simulink model "pro1_21011324"  (R2024b)
settings: Solver=VariableStepAuto  StartTime=0.0  StopTime=500  RelTol=1e-3
InitFcn:
  | %% environment Parameter
  | 
  | g = 9.8066;                      %[m s^2]
  | 
  | %% vehicle Parameter
  | 
  | mass = 1.5;                     %[N]
  | Arm_Length = 0.225;              %[m]
  | %% Motor Parameter
  | 
  | rpm2rad = 2 * pi/60 ;
  | rad2rpm = 1 / rpm2rad;
  | 
  | Friction_Coef = 0.0001;         %[N m/s]
  | Inertia = 2.8e-05;              %[kg m^2]
  | Resistance = 0.1170;            %[ohm]
  | K_Torque = 1 / (rpm2rad * 960); %[N m/A]
  | K_Emf = K_Torque;               %[V s/rad]
  | 
  | Tau = (Inertia * Resistance) / (Resistance * Friction_Coef + K_Torque * K_Emf);
  | 
  | ks = K_Torque / (Resistance * Friction_Coef + K_Torque * K_Emf);
  | 
  | Trust_Coef = 1.1768e-05;        %[N s^2]
  | Drag_Coef = 1.8542e-07;         %[N  m s^2]
  | Hovering_Speed = sqrt((mass * g)/(4 * Trust_Coef));
  | 
  | kp = 0.011;
  | 
  | K1_ALT = 2.1;
  | K2_ALT = 0.7142;
  | 
  | K1_POS = 1.26;
  | K2_POS = 0.4286;
  | 
  | 
  | %waypoint flight
  | wp_1=[0; 0; 80];     %충무관 [m]
  | wp_2=[-564.04; -102.42; 80 ]; % 순리[m]
  | wp_3=[-3714.7; 689.55; 80]; %잠실유람선터미널 [m]
  | wp_home=[0; 0; 50];
libraries: simulink_extras x2, simulink x1, hdlsllib x1
settings Model: Creator=정욱  LastModifiedBy=HOME
settings ConfigComp: CovBoundaryAbsTol=1.0e-5

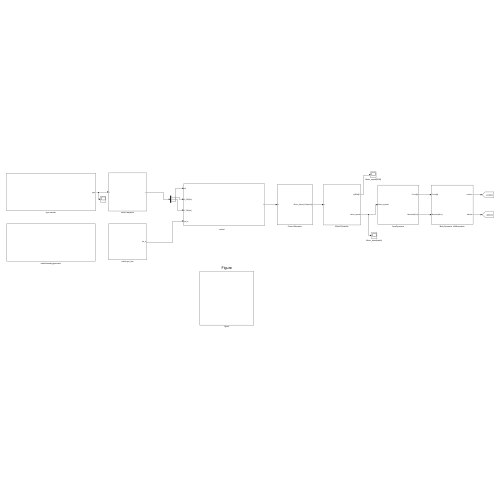
[thumbnail: Simulink's stored preview of the top-level diagram]
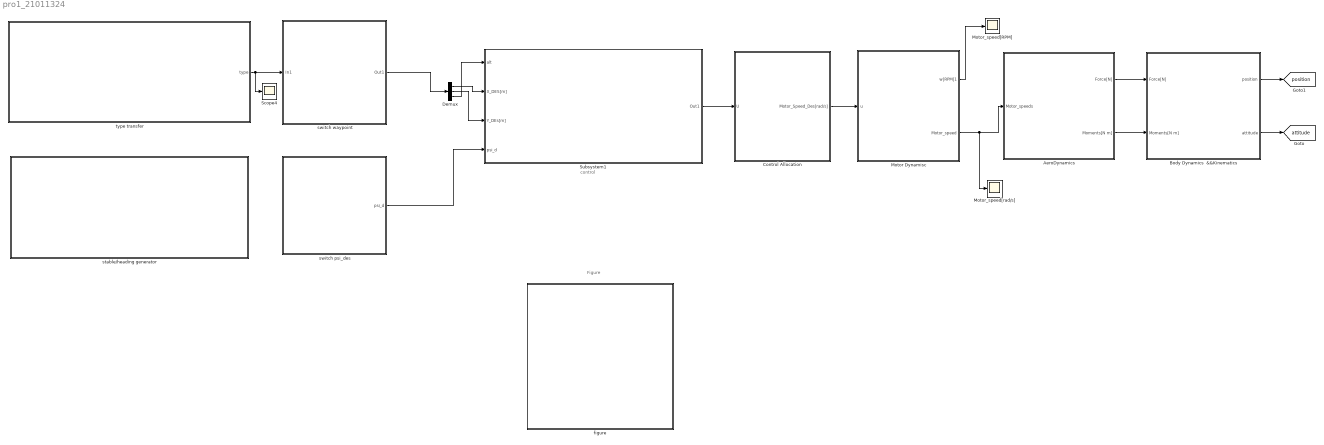
== system pro1_21011324 ==
  note: Figure
  note: control
  AeroDynamics : Subsystem
  Body Dynamics  &&Kinematics : Subsystem
  Control Allocation : Subsystem
  Demux : Demux  Outputs=3
  Motor Dynamisc : Subsystem
  Motor_speed[RPM] : Scope
  Motor_speed[rad/s] : Scope
  Scope4 : Scope
  Subsystem1 : Subsystem
  figure : Subsystem
  stable/heading generator : Subsystem
  switch psi_des : Subsystem
  switch waypoint : Subsystem
  type transfer : Subsystem
  tag scope: attitude=global, position=global
  wires:
  Motor Dynamisc/1(w[RPM]1) -> Motor_speed[RPM]/1
  Motor Dynamisc/2(Motor_speed) -> AeroDynamics/1(Motor_speeds), Motor_speed[rad/s]/1
  Body Dynamics  &&Kinematics/2(attitude) -> [attitude]
  Body Dynamics  &&Kinematics/1(position) -> [position]
  AeroDynamics/1(Force[N]) -> Body Dynamics  &&Kinematics/1(Force[N])
  AeroDynamics/2(Moments[N m]) -> Body Dynamics  &&Kinematics/2(Moments[N m])
  Control Allocation/1(Motor_Speed_Des[rad/s]) -> Motor Dynamisc/1(u)
  Subsystem1/1(Out1) -> Control Allocation/1(U)
  Demux/1 -> Subsystem1/2(X_DES[m])
  Demux/2 -> Subsystem1/3(Y_DEs[m])
  Demux/3 -> Subsystem1/1(alt)
  type transfer/1(type) -> Scope4/1, switch waypoint/1(In1)
  switch waypoint/1(Out1) -> Demux/1
  switch psi_des/1(psi_d) -> Subsystem1/4(psi_d)

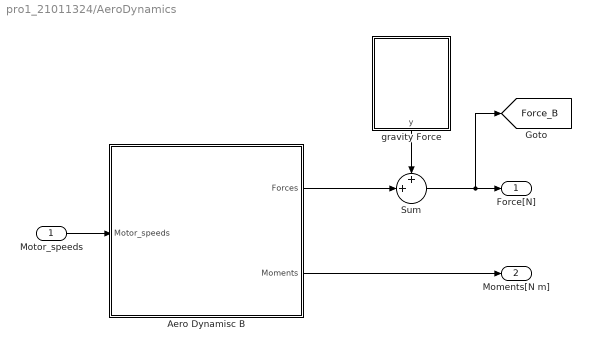
== system pro1_21011324/AeroDynamics ==
  Motor_speeds : Inport
  Aero Dynamisc B : MATLAB Function  TreatAsAtomicUnit=on
  Sum : Sum  Inputs=++|
  "gravity Force " : Subsystem
  Force[N] : Outport
  Moments[N m] : Outport  Port=2
  tag scope: Force_B=global
  wires:
  Aero Dynamisc B/1(Forces) -> Sum/2
  "gravity Force "/1(y) -> Sum/1
  Aero Dynamisc B/2(Moments) -> Moments[N m]/1
  Motor_speeds/1 -> Aero Dynamisc B/1(Motor_speeds)
  Sum/1 -> Force[N]/1, [Force_B]

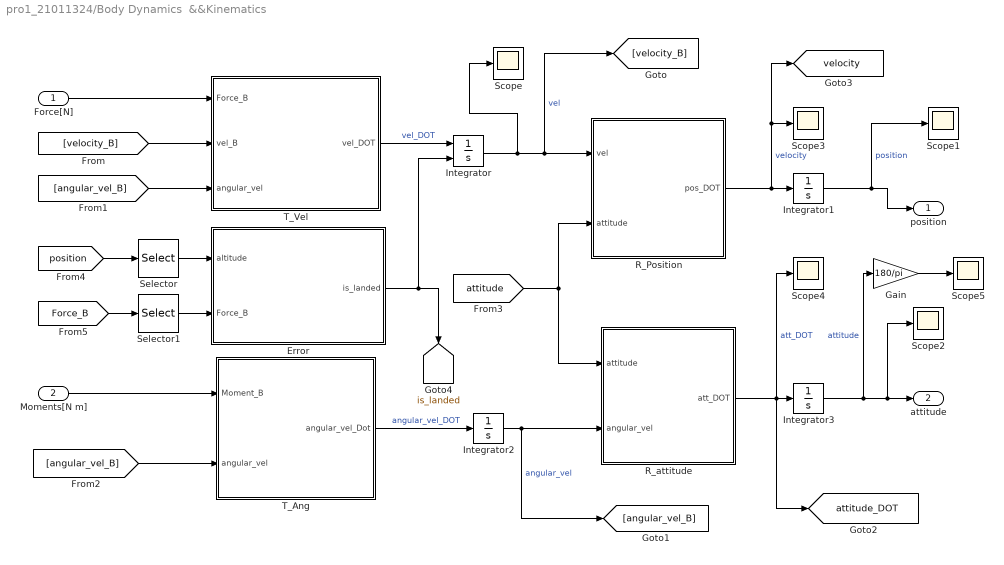
== system pro1_21011324/Body Dynamics  &&Kinematics ==
  Force[N] : Inport
  Moments[N m] : Inport  Port=2
  Error : MATLAB Function  TreatAsAtomicUnit=on
  Gain : Gain  Gain=180/pi
  Integrator : Integrator  ExternalReset=level hold  InitialCondition=[0;0;0]
  Integrator1 : Integrator  InitialCondition=[0;0;0]  LimitOutput=on  UpperSaturationLimit=[inf;inf;0]  LowerSaturationLimit=[-inf;-inf;-inf]  ZeroCross=off
  Integrator2 : Integrator  InitialCondition=[0;0;0]
  Integrator3 : Integrator  InitialCondition=[0;0;0]  WrapState=on
  R_Position : MATLAB Function  TreatAsAtomicUnit=on
  R_attitude : MATLAB Function  TreatAsAtomicUnit=on
  Scope{,1..5} (6 alike) : Scope
  Selector : Selector  InputPortWidth=3  IndexOptions=Index vector (dialog)  Indices=[3]  OutputSizes=1
  Selector1 : Selector  InputPortWidth=3  IndexOptions=Index vector (dialog)  Indices=[3]  OutputSizes=1
  T_Ang : MATLAB Function  TreatAsAtomicUnit=on
  T_Vel : MATLAB Function  TreatAsAtomicUnit=on
  position : Outport
  attitude : Outport  Port=2
  tag scope: attitude_DOT=global, is_landed=global, velocity=global
  wires:
  Force[N]/1 -> T_Vel/1(Force_B)
  Moments[N m]/1 -> T_Ang/1(Moment_B)
  T_Vel/1(vel_DOT) -> Integrator/1  "vel_DOT"
  Integrator/1 -> [velocity_B], R_Position/1(vel), Scope/1  "vel"
  R_Position/1(pos_DOT) -> [velocity], Scope3/1, Integrator1/1  "velocity"
  Integrator1/1 -> Scope1/1, position/1  "position"
  T_Ang/1(angular_vel_Dot) -> Integrator2/1  "angular_vel_DOT"
  Integrator2/1 -> R_attitude/2(angular_vel), [angular_vel_B]  "angular_vel"
  R_attitude/1(att_DOT) -> Scope4/1, [attitude_DOT], Integrator3/1  "att_DOT"
  Integrator3/1 -> Gain/1, Scope2/1, attitude/1  "attitude"
  [velocity_B] -> T_Vel/2(vel_B)
  [angular_vel_B] -> T_Vel/3(angular_vel)
  [angular_vel_B] -> T_Ang/2(angular_vel)
  [attitude] -> R_Position/2(attitude), R_attitude/1(attitude)
  [position] -> Selector/1
  [Force_B] -> Selector1/1
  Selector1/1 -> Error/2(Force_B)
  Selector/1 -> Error/1(altitude)
  Error/1(is_landed) -> [is_landed], Integrator/2
  Gain/1 -> Scope5/1

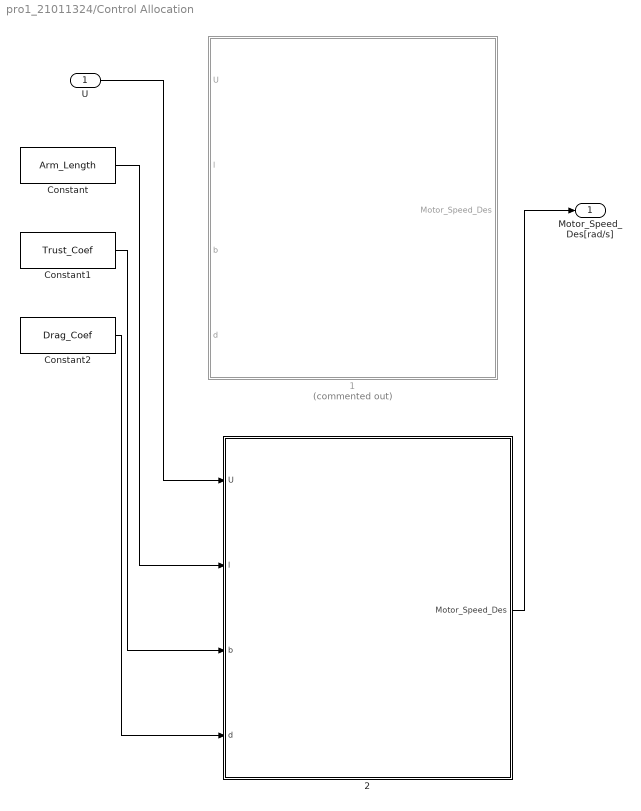
== system pro1_21011324/Control Allocation ==
  U : Inport
  1 : MATLAB Function  Commented=on  TreatAsAtomicUnit=on
  2 : MATLAB Function  TreatAsAtomicUnit=on
  Constant : Constant  Value=Arm_Length
  Constant1 : Constant  Value=Trust_Coef
  Constant2 : Constant  Value=Drag_Coef
  Motor_Speed_Des[rad/s] : Outport
  wires:
  U/1 -> 2/1(U)
  Constant/1 -> 2/2(l)
  Constant1/1 -> 2/3(b)
  Constant2/1 -> 2/4(d)
  2/1(Motor_Speed_Des) -> Motor_Speed_Des[rad/s]/1

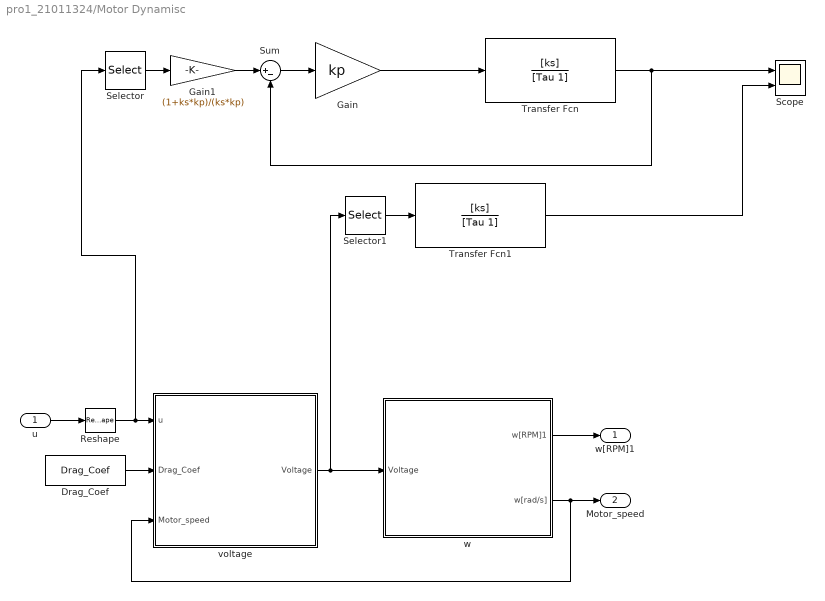
== system pro1_21011324/Motor Dynamisc ==
  u : Inport
  Drag_Coef : Constant  Value=Drag_Coef
  Gain : Gain  Gain=kp
  Gain1 : Gain  Gain=(1+ks*kp)/(ks*kp)
  Reshape : Reshape  OutputDimensionality=Column vector (2-D)
  Scope : Scope  NumInputPorts=2
  Selector : Selector  InputPortWidth=4  IndexOptions=Index vector (dialog)  Indices=1  OutputSizes=1
  Selector1 : Selector  InputPortWidth=4  IndexOptions=Index vector (dialog)  Indices=1  OutputSizes=1
  Sum : Sum  Inputs=|+-
  Transfer Fcn : TransferFcn  Numerator=[ks]  Denominator=[Tau 1]
  Transfer Fcn1 : TransferFcn  Numerator=[ks]  Denominator=[Tau 1]
  voltage : MATLAB Function  TreatAsAtomicUnit=on
  w : Subsystem
  w[RPM]1 : Outport
  Motor_speed : Outport  Port=2
  wires:
  voltage/1(Voltage) -> Selector1/1, w/1(Voltage)
  w/2(w[rad/s]) -> voltage/3(Motor_speed), Motor_speed/1
  u/1 -> Reshape/1
  Drag_Coef/1 -> voltage/2(Drag_Coef)
  w/1(w[RPM]1) -> w[RPM]1/1
  Reshape/1 -> Selector/1, voltage/1(u)
  Selector1/1 -> Transfer Fcn1/1
  Sum/1 -> Gain/1
  Gain/1 -> Transfer Fcn/1
  Transfer Fcn/1 -> Scope/1, Sum/2
  Transfer Fcn1/1 -> Scope/2
  Gain1/1 -> Sum/1
  Selector/1 -> Gain1/1

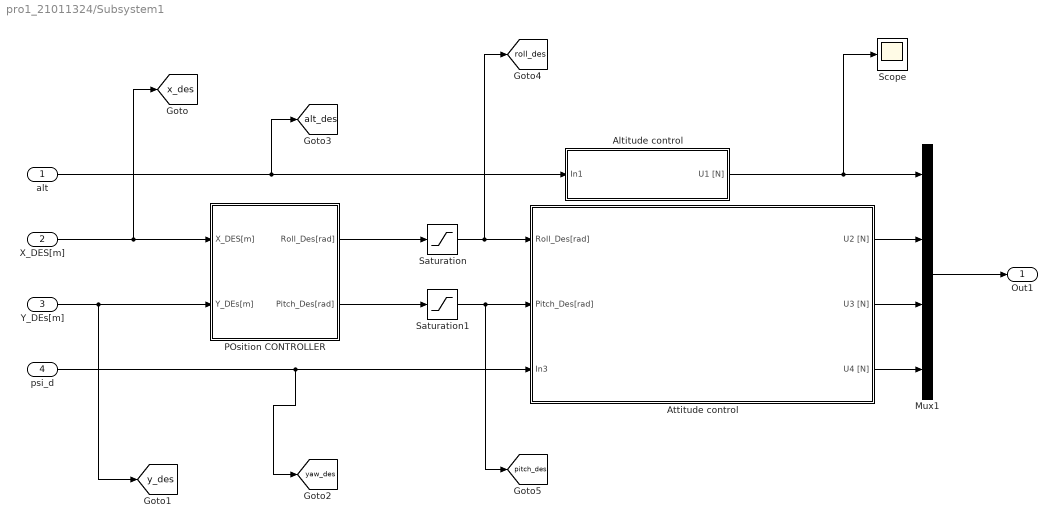
== system pro1_21011324/Subsystem1 ==
  alt : Inport
  X_DES[m] : Inport  Port=2
  Y_DEs[m] : Inport  Port=3
  psi_d : Inport  Port=4
  Altitude control : Subsystem
  Attitude control : Subsystem
  Mux1 : Mux
  POsition CONTROLLER : Subsystem
  Saturation : Saturate  UpperLimit=deg2rad(30)  LowerLimit=-deg2rad(30)
  Saturation1 : Saturate  UpperLimit=deg2rad(30)  LowerLimit=-deg2rad(30)
  Scope : Scope
  Out1 : Outport
  tag scope: alt_des=global, pitch_des=global, roll_des=global, x_des=global, y_des=global, yaw_des=global
  wires:
  Attitude control/3(U4 [N]) -> Mux1/4
  Attitude control/1(U2 [N]) -> Mux1/2
  Saturation/1 -> [roll_des], Attitude control/1(Roll_Des[rad])
  Altitude control/1(U1 [N]) -> Scope/1, Mux1/1
  POsition CONTROLLER/1(Roll_Des[rad]) -> Saturation/1
  Saturation1/1 -> [pitch_des], Attitude control/2(Pitch_Des[rad])
  POsition CONTROLLER/2(Pitch_Des[rad]) -> Saturation1/1
  Attitude control/2(U3 [N]) -> Mux1/3
  Y_DEs[m]/1 -> POsition CONTROLLER/2(Y_DEs[m]), [y_des]
  psi_d/1 -> [yaw_des], Attitude control/3(In3)
  X_DES[m]/1 -> POsition CONTROLLER/1(X_DES[m]), [x_des]
  alt/1 -> [alt_des], Altitude control/1(In1)
  Mux1/1 -> Out1/1

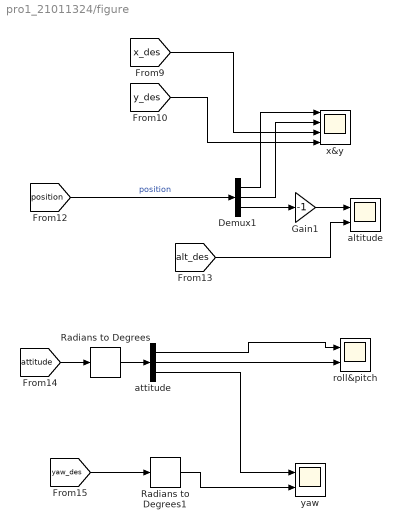
== system pro1_21011324/figure ==
  Demux1 : Demux  Outputs=3
  Gain1 : Gain  Gain=-1
  Radians to Degrees : simulink_extras/Transformations/Radians to Degrees
  Radians to Degrees1 : simulink_extras/Transformations/Radians to Degrees
  altitude : Scope  NumInputPorts=2
  attitude : Demux  Outputs=3
  roll&pitch : Scope  NumInputPorts=2
  x&y : Scope  NumInputPorts=4
  yaw : Scope  NumInputPorts=2
  wires:
  [position] -> Demux1/1  "position"
  Gain1/1 -> altitude/1
  [attitude] -> Radians to Degrees/1
  Demux1/2 -> x&y/2
  [x_des] -> x&y/3
  Demux1/3 -> Gain1/1
  attitude/3 -> yaw/1
  [alt_des] -> altitude/2
  [yaw_des] -> Radians to Degrees1/1
  [y_des] -> x&y/4
  Demux1/1 -> x&y/1
  attitude/2 -> roll&pitch/2
  attitude/1 -> roll&pitch/1
  Radians to Degrees/1 -> attitude/1
  Radians to Degrees1/1 -> yaw/2

== system pro1_21011324/stable//heading generator ==
  Clock : Clock
  MATLAB Function3 : MATLAB Function  TreatAsAtomicUnit=on  SystemSampleTime=0.1
  Scope : Scope
  Selector1 : Selector  InputPortWidth=3  IndexOptions=Index vector (dialog)  Indices=[1]  OutputSizes=1
  Selector2 : Selector  InputPortWidth=3  IndexOptions=Index vector (dialog)  Indices=[2]  OutputSizes=1
  tag scope: stable=global
  wires:
  Selector2/1 -> MATLAB Function3/2(current_pitch)
  [attitude] -> Selector2/1, Selector1/1
  Clock/1 -> MATLAB Function3/3(clock)
  MATLAB Function3/1(stable) -> Scope/1, [stable]
  Selector1/1 -> MATLAB Function3/1(current_roll)

== system pro1_21011324/switch psi_des ==
  Step : Step  Time=0  After=0  SampleTime=0
  psi_d : Outport
  wires:
  Step/1 -> psi_d/1

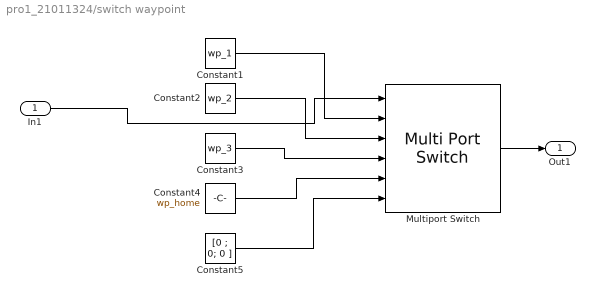
== system pro1_21011324/switch waypoint ==
  In1 : Inport
  Constant1 : Constant  Value=wp_1
  Constant2 : Constant  Value=wp_2
  Constant3 : Constant  Value=wp_3
  Constant4 : Constant  Value=wp_home
  Constant5 : Constant  Value=[0 ; 0; 0 ]
  Multiport Switch : MultiPortSwitch  DataPortOrder=Zero-based contiguous  Inputs=5  DataPortIndices={0,2,4,6,8}  zeroidx=on  SaturateOnIntegerOverflow=off  InputSameDT=off
  Out1 : Outport
  wires:
  Constant2/1 -> Multiport Switch/3
  Constant4/1 -> Multiport Switch/5
  In1/1 -> Multiport Switch/1
  Constant5/1 -> Multiport Switch/6
  Constant3/1 -> Multiport Switch/4
  Constant1/1 -> Multiport Switch/2
  Multiport Switch/1 -> Out1/1

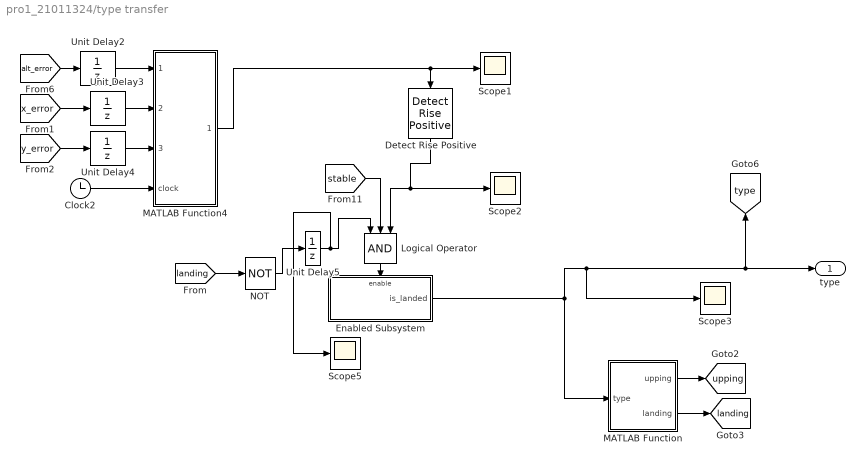
== system pro1_21011324/type transfer ==
  Clock2 : Clock
  Detect Rise Positive : simulink/Logic and Bit Operations/Detect Rise Positive  vinit=0  OutDataTypeStr=boolean
  Enabled Subsystem : Subsystem  TreatAsAtomicUnit=on
  Logical Operator : Logic  Inputs=3  AllPortsSameDT=off  OutDataTypeStr=boolean
  MATLAB Function : MATLAB Function  TreatAsAtomicUnit=on
  MATLAB Function4 : MATLAB Function  TreatAsAtomicUnit=on  SystemSampleTime=0.01
  NOT : Logic  Operator=NOT  IconShape=distinctive  AllPortsSameDT=off  OutDataTypeStr=boolean
  Scope{1..3,5} (4 alike) : Scope
  Unit Delay{2..5} (4 alike) : UnitDelay  SampleTime=-1  HasFrameUpgradeWarning=on
  type : Outport
  tag scope: landing=global, type=global, upping=global
  wires:
  [stable] -> Logical Operator/2
  Unit Delay5/1 -> Scope5/1, Logical Operator/1
  [y_error] -> Unit Delay4/1
  MATLAB Function4/1(arrived) -> Scope1/1, Detect Rise Positive/1
  [alt_error] -> Unit Delay2/1
  Enabled Subsystem/1(is_landed) -> type/1, [type], Scope3/1, MATLAB Function/1(type)
  Detect Rise Positive/1 -> Logical Operator/3, Scope2/1
  Clock2/1 -> MATLAB Function4/4(clock)
  [x_error] -> Unit Delay3/1
  MATLAB Function/1(upping) -> [upping]
  MATLAB Function/2(landing) -> [landing]
  Logical Operator/1 -> Enabled Subsystem/Enable
  NOT/1 -> Unit Delay5/1
  Unit Delay4/1 -> MATLAB Function4/3(y_error)
  [landing] -> NOT/1
  Unit Delay3/1 -> MATLAB Function4/2(x_error)
  Unit Delay2/1 -> MATLAB Function4/1(alt_error)

== system pro1_21011324/AeroDynamics/gravity Force  ==
  gravity : Constant  Value=g
  gravity Foce : MATLAB Function  TreatAsAtomicUnit=on
  mass : Constant  Value=mass
  y : Outport
  wires:
  gravity/1 -> gravity Foce/3(g)
  mass/1 -> gravity Foce/2(m)
  [attitude] -> gravity Foce/1(attitude)
  gravity Foce/1(y) -> y/1

== system pro1_21011324/Motor Dynamisc/w ==
  Voltage : Inport
  G(s) : MATLAB Function  TreatAsAtomicUnit=on
  Integrator : Integrator  InitialCondition=[0;0;0;0]
  w[RPM] : Gain  Gain=rad2rpm
  w[RPM]1 : Outport
  w[rad/s] : Outport  Port=2
  wires:
  G(s)/1(Motoer_speed_Dot) -> Integrator/1  "w_dot[rad/s^2]"
  Integrator/1 -> w[rad/s]/1, w[RPM]/1, G(s)/2(Motor_speed)  "w[rad/s]"
  Voltage/1 -> G(s)/1(Voltage)
  w[RPM]/1 -> w[RPM]1/1  "w[RPM]"

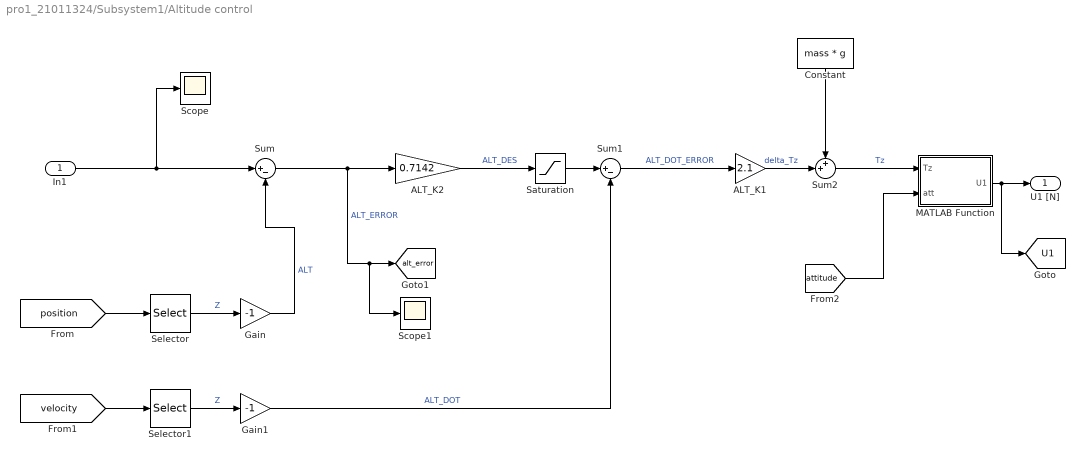
== system pro1_21011324/Subsystem1/Altitude control ==
  In1 : Inport
  ALT_K1 : Gain  Gain=2.1
  ALT_K2 : Gain  Gain=0.7142
  Constant : Constant  Value=mass * g
  Gain : Gain  Gain=-1
  Gain1 : Gain  Gain=-1
  MATLAB Function : MATLAB Function  TreatAsAtomicUnit=on
  Saturation : Saturate  UpperLimit=3  LowerLimit=-1.5
  Scope : Scope
  Scope1 : Scope
  Selector : Selector  InputPortWidth=3  IndexOptions=Index vector (dialog)  Indices=3  OutputSizes=1
  Selector1 : Selector  InputPortWidth=3  IndexOptions=Index vector (dialog)  Indices=3  OutputSizes=1
  Sum : Sum  Inputs=|+-
  Sum1 : Sum  Inputs=|+-
  Sum2 : Sum  Inputs=++|
  U1 [N] : Outport
  tag scope: U1=global, alt_error=global
  wires:
  Constant/1 -> Sum2/1
  [attitude] -> MATLAB Function/2(att)
  Selector/1 -> Gain/1  "Z"
  ALT_K1/1 -> Sum2/2  "delta_Tz"
  [velocity] -> Selector1/1
  Gain1/1 -> Sum1/2  "ALT_DOT"
  Gain/1 -> Sum/2  "ALT"
  [position] -> Selector/1
  Selector1/1 -> Gain1/1  "Z"
  Sum1/1 -> ALT_K1/1  "ALT_DOT_ERROR"
  Sum/1 -> Scope1/1, [alt_error], ALT_K2/1  "ALT_ERROR"
  ALT_K2/1 -> Saturation/1  "ALT_DES"
  Sum2/1 -> MATLAB Function/1(Tz)  "Tz"
  In1/1 -> Sum/1, Scope/1
  MATLAB Function/1(U1) -> [U1], U1 [N]/1
  Saturation/1 -> Sum1/1

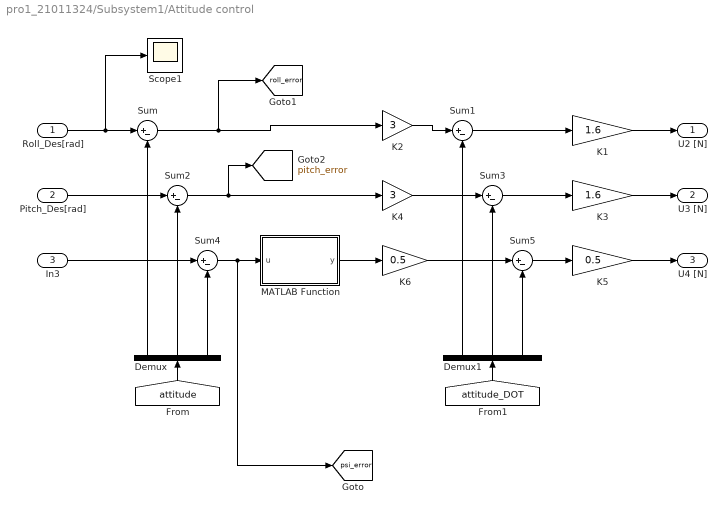
== system pro1_21011324/Subsystem1/Attitude control ==
  Roll_Des[rad] : Inport
  Pitch_Des[rad] : Inport  Port=2
  In3 : Inport  Port=3
  Demux : Demux  Outputs=3
  Demux1 : Demux  Outputs=3
  K1 : Gain  Gain=1.6
  K2 : Gain  Gain=3
  K3 : Gain  Gain=1.6
  K4 : Gain  Gain=3
  K5 : Gain  Gain=0.5
  K6 : Gain  Gain=0.5
  MATLAB Function : MATLAB Function  TreatAsAtomicUnit=on
  Scope1 : Scope
  Sum{,1..5} (6 alike) : Sum  Inputs=|+-
  U2 [N] : Outport
  U3 [N] : Outport  Port=2
  U4 [N] : Outport  Port=3
  tag scope: pitch_error=global, psi_error=global, roll_error=global
  wires:
  Demux/2 -> Sum2/2
  MATLAB Function/1(y) -> K6/1
  Sum1/1 -> K1/1
  Demux1/3 -> Sum5/2
  K6/1 -> Sum5/1
  Sum5/1 -> K5/1
  [attitude] -> Demux/1
  Demux1/1 -> Sum1/2
  K4/1 -> Sum3/1
  Demux/3 -> Sum4/2
  K2/1 -> Sum1/1
  Demux/1 -> Sum/2
  [attitude_DOT] -> Demux1/1
  Sum4/1 -> [psi_error], MATLAB Function/1(u)
  Pitch_Des[rad]/1 -> Sum2/1
  Sum3/1 -> K3/1
  Demux1/2 -> Sum3/2
  Roll_Des[rad]/1 -> Sum/1, Scope1/1
  In3/1 -> Sum4/1
  K3/1 -> U3 [N]/1
  K5/1 -> U4 [N]/1
  K1/1 -> U2 [N]/1
  Sum/1 -> K2/1, [roll_error]
  Sum2/1 -> K4/1, [pitch_error]

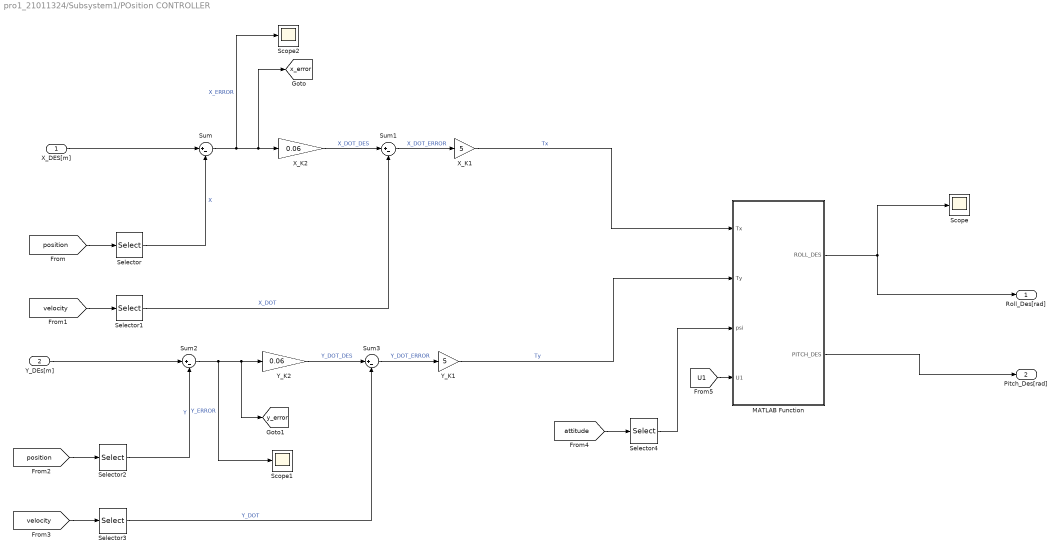
== system pro1_21011324/Subsystem1/POsition CONTROLLER ==
  X_DES[m] : Inport
  Y_DEs[m] : Inport  Port=2
  MATLAB Function : MATLAB Function  TreatAsAtomicUnit=on
  Scope : Scope
  Scope1 : Scope
  Scope2 : Scope
  Selector : Selector  InputPortWidth=3  IndexOptions=Index vector (dialog)  Indices=1  OutputSizes=1
  Selector1 : Selector  InputPortWidth=3  IndexOptions=Index vector (dialog)  Indices=1  OutputSizes=1
  Selector2 : Selector  InputPortWidth=3  IndexOptions=Index vector (dialog)  Indices=2  OutputSizes=1
  Selector3 : Selector  InputPortWidth=3  IndexOptions=Index vector (dialog)  Indices=2  OutputSizes=1
  Selector4 : Selector  InputPortWidth=3  IndexOptions=Index vector (dialog)  Indices=3  OutputSizes=1
  Sum{,1..3} (4 alike) : Sum  Inputs=|+-
  X_K1 : Gain  Gain=5
  X_K2 : Gain  Gain=0.06
  Y_K1 : Gain  Gain=5
  Y_K2 : Gain  Gain=0.06
  Roll_Des[rad] : Outport
  Pitch_Des[rad] : Outport  Port=2
  tag scope: x_error=global, y_error=global
  wires:
  Sum1/1 -> X_K1/1  "X_DOT_ERROR"
  [position] -> Selector/1
  [velocity] -> Selector1/1
  X_K1/1 -> MATLAB Function/1(Tx)  "Tx"
  Sum/1 -> Scope2/1, [x_error], X_K2/1  "X_ERROR"
  Selector/1 -> Sum/2  "X"
  Selector1/1 -> Sum1/2  "X_DOT"
  X_K2/1 -> Sum1/1  "X_DOT_DES"
  X_DES[m]/1 -> Sum/1
  Sum3/1 -> Y_K1/1  "Y_DOT_ERROR"
  [position] -> Selector2/1
  [velocity] -> Selector3/1
  Y_K1/1 -> MATLAB Function/2(Ty)  "Ty"
  Sum2/1 -> Scope1/1, [y_error], Y_K2/1  "Y_ERROR"
  Selector2/1 -> Sum2/2  "Y"
  Selector3/1 -> Sum3/2  "Y_DOT"
  Y_K2/1 -> Sum3/1  "Y_DOT_DES"
  Y_DEs[m]/1 -> Sum2/1
  [attitude] -> Selector4/1
  Selector4/1 -> MATLAB Function/3(psi)
  [U1] -> MATLAB Function/4(U1)
  MATLAB Function/1(ROLL_DES) -> Roll_Des[rad]/1, Scope/1
  MATLAB Function/2(PITCH_DES) -> Pitch_Des[rad]/1

== system pro1_21011324/type transfer/Enabled Subsystem ==
  Enable : EnablePort
  Counter Limited : hdlsllib/Sources/Counter Limited  uplimit=4  tsamp=-1
  is_landed : Outport
  wires:
  Counter Limited/1 -> is_landed/1

== matlab function pro1_21011324/Subsystem1/Attitude control/MATLAB Function ==
  data: u input; y output
function y = fcn(u)

if u < -deg2rad(180)
    y = (deg2rad(360) + u);
elseif u > deg2rad(180)
    y = (-deg2rad(360) + u);

else
    y = u;
end

== matlab function pro1_21011324/Subsystem1/Altitude control/MATLAB Function ==
  data: Tz input; U1 output; att input
function U1 = fcn(Tz, att)

phi = att(1);
theta = att(2);

U1 = Tz / ((cos(phi)) * cos(theta));

== matlab function pro1_21011324/Subsystem1/POsition CONTROLLER/MATLAB Function ==
  data: Tx input; ROLL_DES output; Ty input; psi input; U1 input; PITCH_DES output
function [ROLL_DES, PITCH_DES] = fcn(Tx, Ty, psi, U1)

Txx =  Tx * cos(psi) + Ty * sin(psi);
Tyy = -Tx * sin(psi) + Ty * cos(psi);

ROLL_DES  =  Tyy/U1;
PITCH_DES = -Txx/U1;

== matlab function pro1_21011324/Motor Dynamisc/voltage ==
  data: u input; Drag_Coef input; Voltage output; Motor_speed input
function Voltage = fcn(u, Drag_Coef, Motor_speed)
%% parameter

rpm2rad = 2 * pi/60 ;


Resistance = 0.1170;            %[ohm]

K_Torque = 1 / (rpm2rad * 960); %[N m/A]

K_Emf = K_Torque;               %[V s/rad]

Voltage = K_Emf.*u + (Resistance / K_Torque) * (Drag_Coef .* Motor_speed.^2) ;

end

== matlab function pro1_21011324/type transfer/MATLAB Function4 ==
  settings: updateMethod=DISCRETE
  data: alt_error input; arrived output; x_error input; y_error input; clock input
function arrived = fcn(alt_error, x_error, y_error, clock)

persistent last_trigger_time; % 마지막으로 신호가 발생한 시간 저장

if isempty(last_trigger_time)

last_trigger_time = -3; % 초기값 설정

end


if clock<3

arrived=0;

else

condition = (abs(alt_error) < 1 && abs(x_error) < 10 && abs(y_error) < 10);


if condition && (clock - last_trigger_time >= 1)

arrived = 1;

last_trigger_time = clock;

else

arrived=0;

end

end

end

== matlab function pro1_21011324/type transfer/MATLAB Function ==
  data: type input; upping output; landing output
function [upping, landing] = fcn(type)
upping=double(type)==0;
landing=double(type)==4;

== matlab function pro1_21011324/stable//heading generator/MATLAB Function3 ==
  data: current_roll input; current_pitch input; stable output; clock input
function stable = fcn(current_roll, current_pitch, clock)
    persistent stable_start_time;
    
    if isempty(stable_start_time)
        stable_start_time = -1;
    end

    is_at_level = abs(current_roll) < 0.03 && abs(current_pitch) < 0.03;

    if is_at_level
        if stable_start_time < 0
            stable_start_time = clock; 
        end
        
        if (clock - stable_start_time) >= 2
             stable = 1;
        else
            stable = 0;
        end
    else
        stable_start_time = -1;
        stable = 0;
    end
end

== matlab function pro1_21011324/Motor Dynamisc/w/G(s) ==
  data: Voltage input; Motoer_speed_Dot output; Motor_speed input
function Motoer_speed_Dot = fcn(Voltage, Motor_speed)

%% parameter

rpm2rad = 2 * pi/60 ;

Inertia = 2.8e-05;              %[kg m^2]

Resistance = 0.1170;            %[ohm]

K_Torque = 1 / (rpm2rad * 960); %[N m/A]

K_Emf = K_Torque;               %[V s/rad]
  
Drag_Coef = 1.8542e-07;

%% equation

V_Emf = K_Emf .* Motor_speed; %[Voltage]
Current = (Voltage - V_Emf) / Resistance; %[A] 

Motoer_speed_Dot = (K_Torque * Current - (Drag_Coef .* Motor_speed.^2)) / Inertia; %[rad/s^2]

end

== matlab function pro1_21011324/AeroDynamics/Aero Dynamisc B ==
  data: Motor_speeds input; Forces output; Moments output
function [Forces, Moments]= fcn(Motor_speeds)

%% parameter
Trust_Coef = 1.1768e-05;        %[N s^2]
Drag_Coef = 1.8542e-07;         %[N  m s^2]
Arm_Length = 0.225;             %[N ]

%% equation
Forces = [0;0;-Trust_Coef.*(Motor_speeds(1)^2+Motor_speeds(2)^2+Motor_speeds(3)^2+Motor_speeds(4)^2)];


 % Moments = [Arm_Length*Trust_Coef*(Motor_speeds(4)^2 - Motor_speeds(2)^2);...
 %    Arm_Length*Trust_Coef*(Motor_speeds(1)^2 - Motor_speeds(3)^2);...
 %     Drag_Coef*(-Motor_speeds(1)^2 + Motor_speeds(3)^2 - Motor_speeds(3)^2 + Motor_speeds(4)^2)];

  Moments = [(1/sqrt(2))*Arm_Length*Trust_Coef*(-Motor_speeds(1)^2 + Motor_speeds(2)^2 + Motor_speeds(3)^2 - Motor_speeds(4)^2);...
       (1/sqrt(2))*Arm_Length*Trust_Coef*(Motor_speeds(1)^2 - Motor_speeds(2)^2 + Motor_speeds(3)^2 - Motor_speeds(4)^2);...
       Drag_Coef*(Motor_speeds(1)^2 + Motor_speeds(2)^2 - Motor_speeds(3)^2 - Motor_speeds(4)^2)];
  

end

== matlab function pro1_21011324/AeroDynamics/gravity Force /gravity Foce ==
  data: attitude input; y output; m input; g input
function y = fcn(attitude, m, g)

u = attitude;

R = [cos(u(2))*cos(u(3)) cos(u(2))*sin(u(3)) -sin(u(2))
    sin(u(1))*sin(u(2))*cos(u(3))-cos(u(1))*sin(u(3)) sin(u(1))*sin(u(2))*sin(u(3))+cos(u(1))*cos(u(3)) sin(u(1))*cos(u(2))
    cos(u(1))*sin(u(2))*cos(u(3))+sin(u(1))*sin(u(3)) cos(u(1))*sin(u(2))*sin(u(3))-sin(u(1))*cos(u(3)) cos(u(1))*cos(u(2))];

mg = [0; 0; m*g];

y = R*mg;

== matlab function pro1_21011324/Body Dynamics  &&Kinematics/T_Vel ==
  data: Force_B input; vel_DOT output; vel_B input; angular_vel input
function vel_DOT = fcn(Force_B, vel_B, angular_vel)

m = 1.5; %[kg]

vel_DOT = Force_B / m - cross(angular_vel,vel_B);

== matlab function pro1_21011324/Body Dynamics  &&Kinematics/T_Ang ==
  data: Moment_B input; angular_vel_Dot output; angular_vel input
function angular_vel_Dot = fcn(Moment_B, angular_vel)

I = diag([0.02;0.02;0.025]);

w = angular_vel;


angular_vel_Dot = I^(-1)*(Moment_B - cross(w,I*w));

== matlab function pro1_21011324/Body Dynamics  &&Kinematics/R_Position ==
  data: vel input; pos_DOT output; attitude input
function pos_DOT = fcn(vel, attitude)

u = attitude;

% phi = u(1) 
% theta = u(2) 
% psi = u(3)

R_B2E = [cos(u(2))*cos(u(3)) sin(u(1))*sin(u(2))*cos(u(3))-cos(u(1))*sin(u(3)) cos(u(1))*sin(u(2))*cos(u(3))+sin(u(1))*sin(u(3))
    cos(u(2))*sin(u(3)) sin(u(1))*sin(u(2))*sin(u(3))+cos(u(1))*cos(u(3)) cos(u(1))*sin(u(2))*sin(u(3))-sin(u(1))*cos(u(3))
    -sin(u(2)) sin(u(1))*cos(u(2)) cos(u(1))*cos(u(2))]; 

pos_DOT = R_B2E * vel;

== matlab function pro1_21011324/Body Dynamics  &&Kinematics/R_attitude ==
  data: attitude input; angular_vel input; att_DOT output
function att_DOT = fcn(attitude,angular_vel)

u = attitude;

% phi = u(1) 
% theta = u(2) 
% psi = u(3)

R_B2E = [1 sin(u(1))*tan(u(2)) cos(u(1))*tan(u(2))
0 cos(u(1)) -sin(u(1))
0 sin(u(1))/cos(u(2)) cos(u(1))/cos(u(2))];

att_DOT = R_B2E*angular_vel;

== matlab function pro1_21011324/Body Dynamics  &&Kinematics/Error ==
  data: altitude input; is_landed output; Force_B input
function is_landed = fcn(altitude, Force_B)

is_landed = (altitude >= 0) && (Force_B > 0);

end

== matlab function pro1_21011324/Control Allocation/1 ==
  data: U input; Motor_Speed_Des output; l input; b input; d input
function Motor_Speed_Des = fcn(U, l, b, d)

AC = [b b b b;0 -l*b 0 l*b;l*b 0 -l*b 0;-d d -d d]^(-1);

Motor_Speed_Des_2 = max(AC * U,0);

Motor_Speed_Des = sqrt(Motor_Speed_Des_2);

== matlab function pro1_21011324/Control Allocation/2 ==
  data: U input; Motor_Speed_Des output; l input; b input; d input
function Motor_Speed_Des = fcn(U, l, b, d)

AC = [b b b b;
    -l*b/sqrt(2) l*b/sqrt(2) l*b/sqrt(2) -l*b/sqrt(2);
    l*b/sqrt(2) -l*b/sqrt(2) l*b/sqrt(2) -l*b/sqrt(2);
    d d -d -d]^(-1);

Motor_Speed_Des_2 = max(AC * U,0);

Motor_Speed_Des = sqrt(Motor_Speed_Des_2);
